simulink library "Lib_Common"  (R2014b)
settings: Solver=ode45  StartTime=0.0  StopTime=10.0  RelTol=1e-3
undefined symbols (not defined in the file or in its folder): sigbuilder_block
libraries: simulink x4
settings Model: Creator=Ehang  LastModifiedBy=Ehang

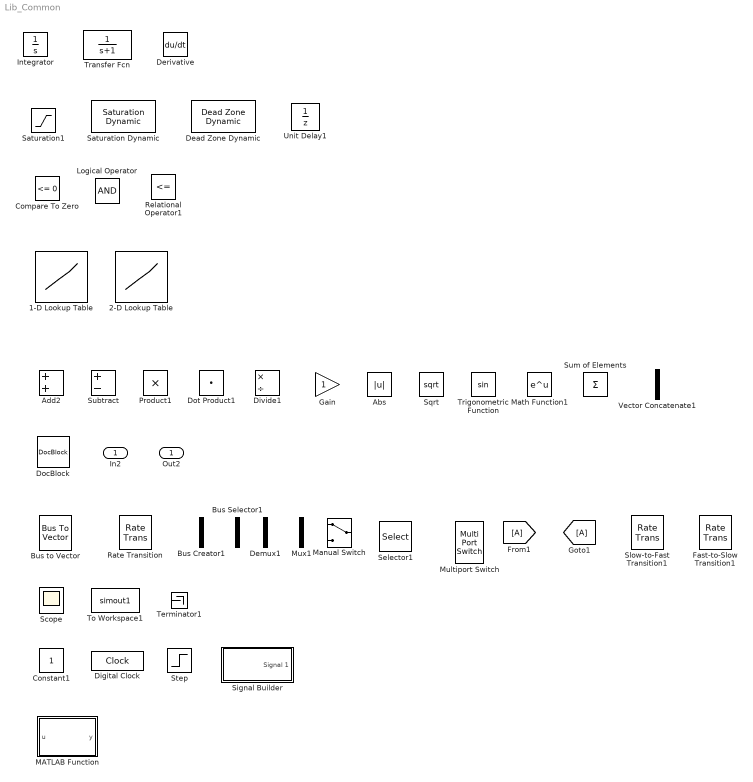
== system Lib_Common ==
  In2 : Inport
  1-D Lookup Table : Lookup_n-D  NumberOfTableDimensions=1  BreakpointsForDimension1=[-5:5]  Table=tanh([-5:5])  InternalRulePriority=Speed  RndMeth=Simplest  InputSameDT=on
  2-D Lookup Table : Lookup_n-D  BreakpointsForDimension1=[1:3]  BreakpointsForDimension2=[1:3]  InternalRulePriority=Speed  RndMeth=Simplest  InputSameDT=on
  Abs : Abs
  Add2 : Sum
  Bus Creator1 : BusCreator  Inputs=3
  Bus Selector1 : BusSelector  OutputSignals=signal1,signal2
  Bus to Vector : BusToVector
  Compare To Zero : simulink/Logic and Bit Operations/Compare To Zero  relop=<=  OutDataTypeStr=boolean
  Constant1 : Constant
  Dead Zone Dynamic : simulink/Discontinuities/Dead Zone Dynamic
  Demux1 : Demux  Outputs=2
  Derivative : Derivative
  Digital Clock : DigitalClock
  Divide1 : Product  Inputs=*/
  DocBlock : simulink/Model-Wide Utilities/DocBlock  DocumentType=Text
      content=|
      | Type your documentation here
  Dot Product1 : DotProduct  InputSameDT=on  OutDataTypeStr=Inherit: Inherit via internal rule
  Fast-to-Slow Transition1 : RateTransition
  Gain : Gain
  Integrator : Integrator
  Logical Operator : Logic  AllPortsSameDT=off  OutDataTypeStr=boolean
  MATLAB Function : MATLAB Function  TreatAsAtomicUnit=on
  Manual Switch : ManualSwitch
  Math Function1 : Math  SaturateOnIntegerOverflow=on
  Multiport Switch : MultiPortSwitch
  Mux1 : Mux  Inputs=3
  Product1 : Product
  Rate Transition : RateTransition
  Relational Operator1 : RelationalOperator  Operator=<=  OutDataTypeStr=boolean
  Saturation Dynamic : simulink/Discontinuities/Saturation Dynamic  OutMin=[]  OutMax=[]  OutDataTypeStr=Inherit: Same as second input  OutDataType=fixdt(1, 16)  OutScaling=2^-10  DoSatur=off
  Saturation1 : Saturate
  Scope : Scope
  Selector1 : Selector  InputPortWidth=3  Indices=[1 3]
  Signal Builder : Subsystem  Tag=STV Subsys  LoadFcn=sigbuilder_block('load');  StartFcn=sigbuilder_block('start');  StopFcn=sigbuilder_block('stop');  ClipboardFcn=sigbuilder_block('clipboard');  mask(Sigbuilder block){}
      mask help: Simulink:masks:SigbuilderBlock_MD
      mask init:
      | if ~strcmp(get_param(bdroot(gcbh),'SimulationStatus'),'stopped') tuvar = sigbuilder_block('maskInit'); end
      settings: CopyFcn=sigbuilder_block('copy');  DeleteFcn=sigbuilder_block('delete');  ModelCloseFcn=sigbuilder_block('modelClose');  PreSaveFcn=sigbuilder_block('preSave');  PauseFcn=sigbuilder_block('pause');  ContinueFcn=sigbuilder_block('continue');  NameChangeFcn=sigbuilder_block('namechange');  OpenFcn=sigbuilder_block('open',[437.6 199.2 550.4 400 ]);  CloseFcn=sigbuilder_block('close');
      mask Display: plot(0, 0, 100, 100,[2, 2, 32, 32, 2], [68, 8, 8, 68, 68],[32, 2], [38, 38], [32, 19, 2],[53, 60, 44], [32, 17, 17, 2],[16, 16, 31, 31]);txt = getActiveGroup(gcbh);text(2, 100, txt,'verticalAlignment', 'top');
  Slow-to-Fast Transition1 : RateTransition
  Sqrt : Sqrt  SaturateOnIntegerOverflow=on
  Step : Step  SampleTime=0
  Subtract : Sum  Inputs=+-
  Sum of Elements : Sum  Inputs=+
  Terminator1 : Terminator
  To Workspace1 : ToWorkspace  VariableName=simout1  SaveFormat=Timeseries  SampleTime=-1
  Transfer Fcn : TransferFcn  Denominator=[1 1]
  Trigonometric Function : Trigonometry
  Unit Delay1 : UnitDelay  SampleTime=-1
  Vector Concatenate1 : Concatenate
  Out2 : Outport

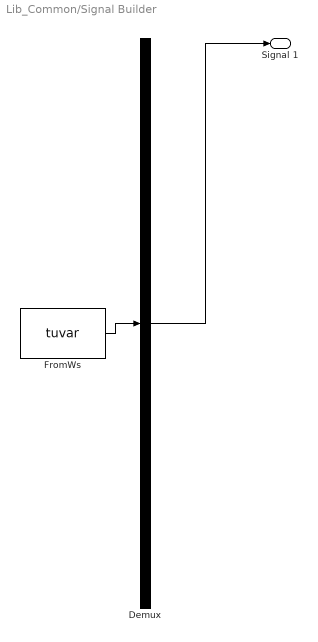
== system Lib_Common/Signal Builder ==
  Demux : Demux  Tag=STV Demux  Outputs=1
  FromWs : FromWorkspace  Tag=STV FromWs  VariableName=tuvar  SampleTime=0
      SigBuilderData=|
      | common.afterFinalStr = 'Extrapolate'
      | common.sampleTime = 0
      | dataSet.timeRange = [0 10]
      | dataSet.name = 'Group 1'
      | sbobj.Groups.Name = 'Group 1'
      | sbobj.Groups.Signals.Name = 'Signal 1'
      | sbobj.Groups.Signals.XData = [0 4 4 6 6 10]
      | sbobj.Groups.Signals.YData = [0 0 1 1 0 0]
  Signal 1 : Outport  Tag=STV Outport
  wires:
  Demux/1 -> Signal 1/1
  FromWs/1 -> Demux/1

== matlab function Lib_Common/MATLAB Function ==
  data: u input; y output
function y = fcn(u)
%#codegen

y = u;
